simulink model "testingCar"  (R2024a)
settings: Solver=VariableStepAuto  StartTime=0.0  StopTime=10.0  RelTol=1e-3
undefined symbols (not defined in the file or in its folder): A0, A1, A2, A3, ended, GND, Single
libraries: raspberrypiBasiclib x12
settings Model: Creator=user  LastModifiedBy=user

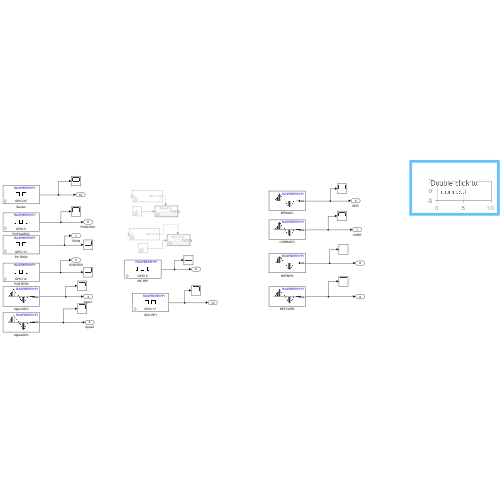
[thumbnail: Simulink's stored preview of the top-level diagram]
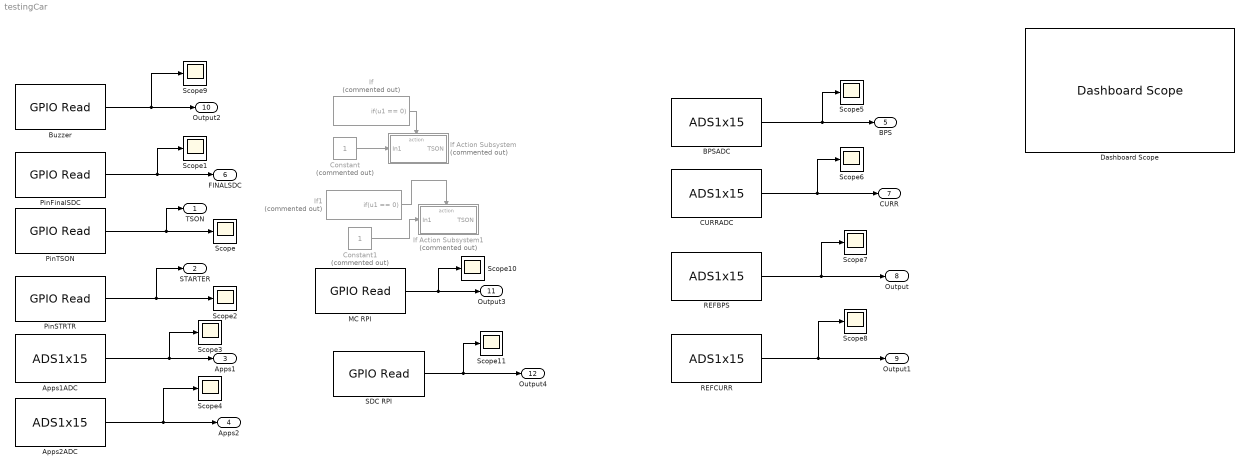
== system testingCar ==
  Apps1ADC : raspberrypiBasiclib/ADS1x15  ADCChip=ADS1115  I2CAddress=0x48  ConversionMode=Single-shot  InputConfiguration=A2 - GND (Single-ended)  GainConfigurationDifferential=+/- 2.048 V  GainConfigurationSingleEnded=1.024 V  DataRateConfigurationADS1015=1600SPS  DataRateConfigurationADS1115=860SPS  SampleTime=0.1  EnableComparatorMode=off  ComparatorMode=Traditional with hysterisis  ComparatorPolarityConfiguration=Active low  ComparatorLatchingConfiguration=Non-latching  ComparatorQueueConfiguration=Assert after 1 conversion  ComparatorLowThresholdADS1015=0  ComparatorLowThresholdADS1115=0  ComparatorHighThresholdADS1015=0  ComparatorHighThresholdADS1115=0
  Apps2ADC : raspberrypiBasiclib/ADS1x15  ADCChip=ADS1115  I2CAddress=0x48  ConversionMode=Single-shot  InputConfiguration=A3 - GND (Single-ended)  GainConfigurationDifferential=+/- 2.048 V  GainConfigurationSingleEnded=1.024 V  DataRateConfigurationADS1015=1600SPS  DataRateConfigurationADS1115=860SPS  SampleTime=0.1  EnableComparatorMode=off  ComparatorMode=Traditional with hysterisis  ComparatorPolarityConfiguration=Active low  ComparatorLatchingConfiguration=Non-latching  ComparatorQueueConfiguration=Assert after 1 conversion  ComparatorLowThresholdADS1015=0  ComparatorLowThresholdADS1115=0  ComparatorHighThresholdADS1015=0  ComparatorHighThresholdADS1115=0
  BPSADC : raspberrypiBasiclib/ADS1x15  ADCChip=ADS1115  I2CAddress=0x49  ConversionMode=Single-shot  InputConfiguration=A1 - GND (Single-ended)  GainConfigurationDifferential=+/- 2.048 V  GainConfigurationSingleEnded=1.024 V  DataRateConfigurationADS1015=1600SPS  DataRateConfigurationADS1115=860SPS  SampleTime=0.1  EnableComparatorMode=off  ComparatorMode=Traditional with hysterisis  ComparatorPolarityConfiguration=Active low  ComparatorLatchingConfiguration=Non-latching  ComparatorQueueConfiguration=Assert after 1 conversion  ComparatorLowThresholdADS1015=0  ComparatorLowThresholdADS1115=0  ComparatorHighThresholdADS1015=0  ComparatorHighThresholdADS1115=0
  Buzzer : raspberrypiBasiclib/GPIO Read  board=Pi Zero 2 W  gpio=25  internalResistor=Off  sampleTime=0.1  direction=Input  blockPlatform=Raspberry Pi
  CURRADC : raspberrypiBasiclib/ADS1x15  ADCChip=ADS1115  I2CAddress=0x49  ConversionMode=Single-shot  InputConfiguration=A0 - GND (Single-ended)  GainConfigurationDifferential=+/- 2.048 V  GainConfigurationSingleEnded=1.024 V  DataRateConfigurationADS1015=1600SPS  DataRateConfigurationADS1115=860SPS  SampleTime=0.1  EnableComparatorMode=off  ComparatorMode=Traditional with hysterisis  ComparatorPolarityConfiguration=Active low  ComparatorLatchingConfiguration=Non-latching  ComparatorQueueConfiguration=Assert after 1 conversion  ComparatorLowThresholdADS1015=0  ComparatorLowThresholdADS1115=0  ComparatorHighThresholdADS1015=0  ComparatorHighThresholdADS1115=0
  Constant : Constant  Commented=on
  Constant1 : Constant  Commented=on
  Dashboard Scope : DashboardScope
  If : If  Commented=on  IfExpression=u1 == 0  ShowElse=off
  If Action Subsystem : Subsystem  Commented=on  TreatAsAtomicUnit=on
  If Action Subsystem1 : Subsystem  Commented=on  TreatAsAtomicUnit=on
  If1 : If  Commented=on  IfExpression=u1 == 0  ShowElse=off
  MC RPI : raspberrypiBasiclib/GPIO Read  board=Pi Zero 2 W  gpio=6  internalResistor=Off  sampleTime=0.1  direction=Input  blockPlatform=Raspberry Pi
  PinFinalSDC : raspberrypiBasiclib/GPIO Read  board=Pi Zero 2 W  gpio=5  internalResistor=Off  sampleTime=0.1  direction=Input  blockPlatform=Raspberry Pi
  PinSTRTR : raspberrypiBasiclib/GPIO Read  board=Pi Zero 2 W  gpio=12  internalResistor=Off  sampleTime=0.1  direction=Input  blockPlatform=Raspberry Pi
  PinTSON : raspberrypiBasiclib/GPIO Read  board=Pi Zero 2 W  gpio=13  internalResistor=Off  sampleTime=0.1  direction=Input  blockPlatform=Raspberry Pi
  REFBPS : raspberrypiBasiclib/ADS1x15  ADCChip=ADS1115  I2CAddress=0x49  ConversionMode=Single-shot  InputConfiguration=A2 - GND (Single-ended)  GainConfigurationDifferential=+/- 2.048 V  GainConfigurationSingleEnded=1.024 V  DataRateConfigurationADS1015=1600SPS  DataRateConfigurationADS1115=860SPS  SampleTime=0.1  EnableComparatorMode=off  ComparatorMode=Traditional with hysterisis  ComparatorPolarityConfiguration=Active low  ComparatorLatchingConfiguration=Non-latching  ComparatorQueueConfiguration=Assert after 1 conversion  ComparatorLowThresholdADS1015=0  ComparatorLowThresholdADS1115=0  ComparatorHighThresholdADS1015=0  ComparatorHighThresholdADS1115=0
  REFCURR : raspberrypiBasiclib/ADS1x15  ADCChip=ADS1115  I2CAddress=0x49  ConversionMode=Single-shot  InputConfiguration=A3 - GND (Single-ended)  GainConfigurationDifferential=+/- 2.048 V  GainConfigurationSingleEnded=1.024 V  DataRateConfigurationADS1015=1600SPS  DataRateConfigurationADS1115=860SPS  SampleTime=0.1  EnableComparatorMode=off  ComparatorMode=Traditional with hysterisis  ComparatorPolarityConfiguration=Active low  ComparatorLatchingConfiguration=Non-latching  ComparatorQueueConfiguration=Assert after 1 conversion  ComparatorLowThresholdADS1015=0  ComparatorLowThresholdADS1115=0  ComparatorHighThresholdADS1015=0  ComparatorHighThresholdADS1115=0
  SDC RPI : raspberrypiBasiclib/GPIO Read  board=Pi Zero 2 W  gpio=17  internalResistor=Off  sampleTime=0.1  direction=Input  blockPlatform=Raspberry Pi
  Scope{,1..11} (12 alike) : Scope
  TSON : Outport
  STARTER : Outport  Port=2
  Apps1 : Outport  Port=3
  Apps2 : Outport  Port=4
  BPS : Outport  Port=5
  FINALSDC : Outport  Port=6
  CURR : Outport  Port=7
  Output : Outport  Port=8
  Output1 : Outport  Port=9
  Output2 : Outport  Port=10
  Output3 : Outport  Port=11
  Output4 : Outport  Port=12
  wires:
  If/1 -> If Action Subsystem/Action
  Constant/1 -> If Action Subsystem/1(In1)
  If1/1 -> If Action Subsystem1/Action
  Constant1/1 -> If Action Subsystem1/1(In1)
  Apps1ADC/1 -> Scope3/1, Apps1/1
  PinFinalSDC/1 -> Scope1/1, FINALSDC/1
  Apps2ADC/1 -> Scope4/1, Apps2/1
  BPSADC/1 -> Scope5/1, BPS/1
  PinTSON/1 -> TSON/1, Scope/1
  PinSTRTR/1 -> STARTER/1, Scope2/1
  CURRADC/1 -> Scope6/1, CURR/1
  REFBPS/1 -> Scope7/1, Output/1
  REFCURR/1 -> Scope8/1, Output1/1
  Buzzer/1 -> Scope9/1, Output2/1
  MC RPI/1 -> Scope10/1, Output3/1
  SDC RPI/1 -> Scope11/1, Output4/1

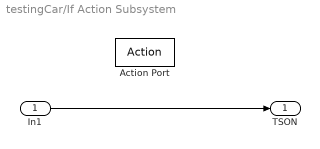
== system testingCar/If Action Subsystem ==
  In1 : Inport
  Action Port : ActionPort  ActionPortLabel=if(u1 == 0)
  TSON : Outport
  wires:
  In1/1 -> TSON/1

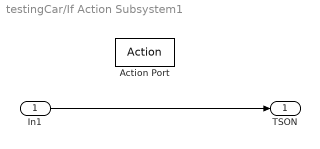
== system testingCar/If Action Subsystem1 ==
  In1 : Inport
  Action Port : ActionPort  ActionPortLabel=if(u1 == 0)
  TSON : Outport
  wires:
  In1/1 -> TSON/1
